simulink model "controladorPV2"  (Simulink 8.3)
settings: Solver=ode45  StartTime=0.0  StopTime=500  MaxStep=0.03  MinStep=0.01  RelTol=1e-3
libraries: dspsigops x8
settings Model: Creator=Daniel  LastModifiedBy=Lab Automática
settings SolverCC: InitialStep=0.01
settings OptimizationCC: ExpressionDepthLimit=2147483647
settings DebuggingCC: FcnCallInpInsideContextMsg=UseLocalSettings

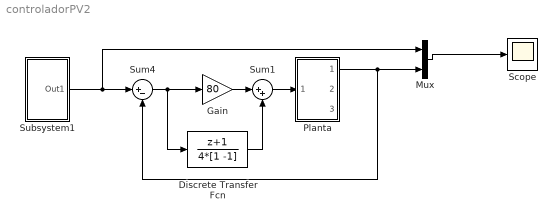
== system controladorPV2 ==
  Discrete Transfer Fcn : DiscreteTransferFcn  Numerator=[1 1]  Denominator=4*[1 -1]  SampleTime=.1
  Gain : Gain  Gain=80
  Mux : Mux  Inputs=2
  Planta : Subsystem
  Scope : Scope
      settings: TimeRange=1000  YMin=10  YMax=40  SaveName=ScopeData2
  Subsystem1 : Subsystem
  Sum1 : Sum  Inputs=|++
  Sum4 : Sum  Inputs=|+-  SampleTime=0.1
  wires:
  Planta/1(Out1) -> Mux/2, Sum4/2
  Mux/1 -> Scope/1
  Sum4/1 -> Discrete Transfer Fcn/1, Gain/1
  Subsystem1/1(Out1) -> Sum4/1, Mux/1
  Gain/1 -> Sum1/1
  Sum1/1 -> Planta/1(In1)
  Discrete Transfer Fcn/1 -> Sum1/2

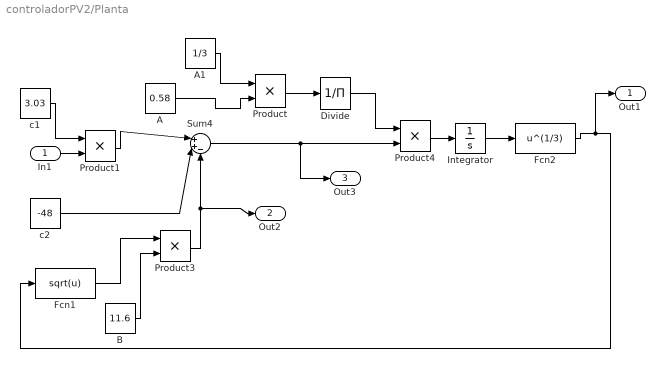
== system controladorPV2/Planta ==
  In1 : Inport
  A : Constant  Value=0.58
  A1 : Constant  Value=1/3
  B : Constant  Value=11.6
  Divide : Product  Inputs=/
  Fcn1 : Fcn  Expr=sqrt(u)  SampleTime=0.1
  Fcn2 : Fcn  Expr=u^(1/3)  SampleTime=0.1
  Integrator : Integrator  InitialCondition=25*25*25  LowerSaturationLimit=0.1
  Product : Product  Inputs=**  RndMeth=Zero
  Product1 : Product  SampleTime=0.1  RndMeth=Zero
  Product3 : Product  SampleTime=0.1  RndMeth=Zero
  Product4 : Product  SampleTime=0.1  RndMeth=Zero
  Sum4 : Sum  Inputs=|++-
  c1 : Constant  Value=3.03
  c2 : Constant  Value=-48
  Out1 : Outport
  Out2 : Outport  Port=2
  Out3 : Outport  Port=3
  wires:
  c1/1 -> Product1/1
  Product1/1 -> Sum4/1
  c2/1 -> Sum4/2
  Fcn1/1 -> Product3/1
  B/1 -> Product3/2
  Product3/1 -> Sum4/3, Out2/1
  Sum4/1 -> Product4/2, Out3/1
  Divide/1 -> Product4/1
  Product/1 -> Divide/1
  Product4/1 -> Integrator/1
  In1/1 -> Product1/2
  A/1 -> Product/2
  A1/1 -> Product/1
  Integrator/1 -> Fcn2/1
  Fcn2/1 -> Fcn1/1, Out1/1

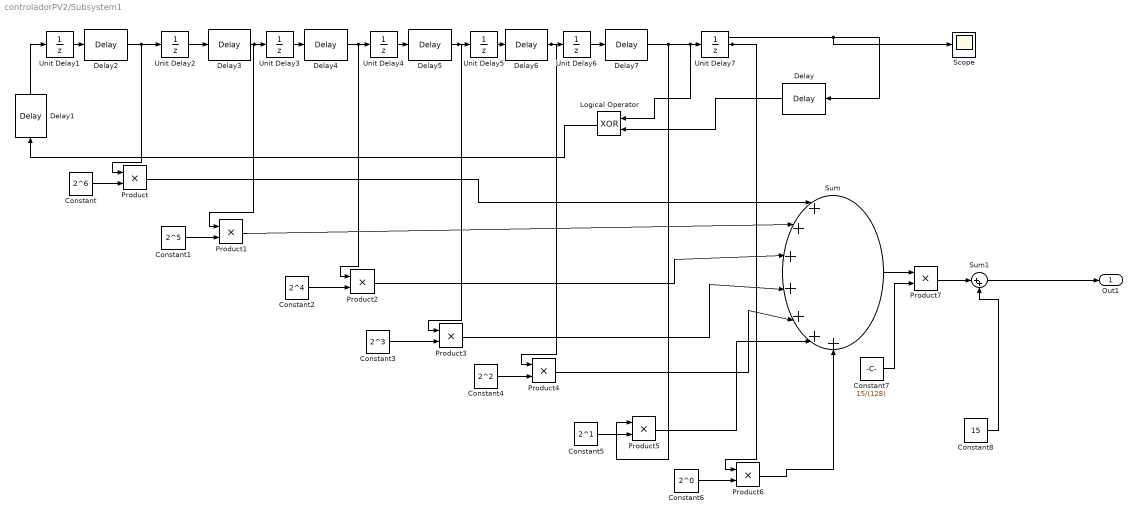
== system controladorPV2/Subsystem1 ==
  Constant : Constant  Value=2^6
  Constant1 : Constant  Value=2^5
  Constant2 : Constant  Value=2^4
  Constant3 : Constant  Value=2^3
  Constant4 : Constant  Value=2^2
  Constant5 : Constant  Value=2^1
  Constant6 : Constant  Value=2^0
  Constant7 : Constant  Value=15/(128)
  Constant8 : Constant  Value=15
  Delay{,1..7} (8 alike) : dspsigops/Delay  InputProcessing=Columns as channels (frame based)  dly_unit=Samples  delay=800  ic_detail=off  dif_ic_for_ch=off  dif_ic_for_dly=off  ic=1  reset_popup=None
  Logical Operator : Logic  Operator=XOR  AllPortsSameDT=off  OutDataTypeStr=boolean
  Product{,1..7} (8 alike) : Product  RndMeth=Zero
  Scope : Scope
  Sum : Sum  Inputs=|+++++++
  Sum1 : Sum  Inputs=|++  SampleTime=0.1
  Unit Delay{1..7} (7 alike) : UnitDelay  InitialCondition=1  SampleTime=0.1
  Out1 : Outport
  wires:
  Unit Delay1/1 -> Delay2/1
  Unit Delay2/1 -> Delay3/1
  Unit Delay3/1 -> Delay4/1
  Unit Delay4/1 -> Delay5/1
  Unit Delay5/1 -> Delay6/1
  Logical Operator/1 -> Delay1/1
  Unit Delay6/1 -> Delay7/1
  Unit Delay7/1 -> Delay/1, Scope/1, Product6/1
  Product/1 -> Sum/1
  Product1/1 -> Sum/2
  Product2/1 -> Sum/3
  Product3/1 -> Sum/4
  Product4/1 -> Sum/5
  Product5/1 -> Sum/6
  Product6/1 -> Sum/7
  Constant/1 -> Product/2
  Constant1/1 -> Product1/2
  Constant2/1 -> Product2/2
  Constant3/1 -> Product3/2
  Constant6/1 -> Product6/2
  Constant5/1 -> Product5/2
  Constant4/1 -> Product4/2
  Sum/1 -> Product7/1
  Constant7/1 -> Product7/2
  Constant8/1 -> Sum1/2
  Product7/1 -> Sum1/1
  Sum1/1 -> Out1/1
  Delay/1 -> Logical Operator/2
  Delay7/1 -> Logical Operator/1, Unit Delay7/1, Product5/1
  Delay2/1 -> Unit Delay2/1, Product/1
  Delay3/1 -> Product1/1, Unit Delay3/1
  Delay4/1 -> Unit Delay4/1, Product2/1
  Delay5/1 -> Product3/1, Unit Delay5/1
  Delay6/1 -> Product4/1, Unit Delay6/1
  Delay1/1 -> Unit Delay1/1
